simulink model "Ejercicio18_20_02_17"  (R2013a)
settings: Solver=ode45  StartTime=0.0  StopTime=100  RelTol=1e-3
settings Model: Creator=Miguel  LastModifiedBy=Miguel

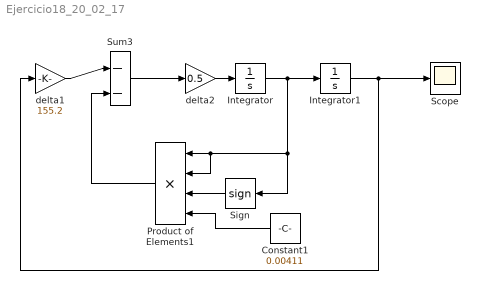
== system Ejercicio18_20_02_17 ==
  Constant1 : Constant  Value=0.00411
  Integrator : Integrator
  Integrator1 : Integrator  InitialCondition=1
  Product of Elements1 : Product  Inputs=4
  Scope : Scope
      settings: ShowLegends=on  TimeRange=10
  Sign : Signum
  Sum3 : Sum  Inputs=|--
  delta1 : Gain  Gain=155.2
  delta2 : Gain  Gain=0.5
  wires:
  Sum3/1 -> delta2/1
  Integrator1/1 -> Scope/1, delta1/1
  Integrator/1 -> Sign/1, Product of Elements1/2, Product of Elements1/1, Integrator1/1
  delta1/1 -> Sum3/1
  Sign/1 -> Product of Elements1/3
  Constant1/1 -> Product of Elements1/4
  Product of Elements1/1 -> Sum3/2
  delta2/1 -> Integrator/1
